simulink library "FIN_MDL"  (R2015a)
settings: Solver=ode45  StartTime=0.0  StopTime=10.0  RelTol=1e-3
undefined symbols (not defined in the file or in its folder): FIN, VAF
libraries: simulink x4
settings Model: Creator=Andrew  LastModifiedBy=Andrew

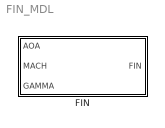
== system FIN_MDL ==
  FIN : Subsystem  mask{FIN=FIN}
      mask prompts: FIN "INPUT  PARAMETERS"

== system FIN_MDL/FIN ==
  AOA : Inport
  MACH : Inport  Port=2
  GAMMA : Inport  Port=3
  Bus Creator : BusCreator  Inputs=5
  FIN_SET_MDL : Subsystem
  FIN : Outport
  wires:
  AOA/1 -> FIN_SET_MDL/1(AOA)
  MACH/1 -> FIN_SET_MDL/2(MACH)
  GAMMA/1 -> FIN_SET_MDL/3(GAMMA)
  FIN_SET_MDL/2(FIN_CN_ALPHA) -> Bus Creator/2  "CN_ALPHA"
  FIN_SET_MDL/1(FIN_CP) -> Bus Creator/1  "CP"
  Bus Creator/1 -> FIN/1
  FIN_SET_MDL/5(FIN_REF_AREA) -> Bus Creator/5  "REF_AREA"
  FIN_SET_MDL/4(FIN_CD) -> Bus Creator/4  "CD"
  FIN_SET_MDL/3(FIN_CN_ALPHA_1) -> Bus Creator/3  "CN_ALPHA_1"

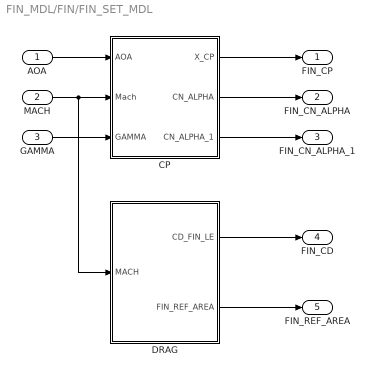
== system FIN_MDL/FIN/FIN_SET_MDL ==
  AOA : Inport
  MACH : Inport  Port=2
  GAMMA : Inport  Port=3
  CP : Subsystem
  DRAG : Subsystem
  FIN_CP : Outport
  FIN_CN_ALPHA : Outport  Port=2
  FIN_CN_ALPHA_1 : Outport  Port=3
  FIN_CD : Outport  Port=4
  FIN_REF_AREA : Outport  Port=5
  wires:
  CP/1(X_CP) -> FIN_CP/1
  CP/2(CN_ALPHA) -> FIN_CN_ALPHA/1
  DRAG/1(CD_FIN_LE) -> FIN_CD/1
  DRAG/2(FIN_REF_AREA) -> FIN_REF_AREA/1
  AOA/1 -> CP/1(AOA)
  GAMMA/1 -> CP/3(GAMMA)
  MACH/1 -> DRAG/1(MACH), CP/2(Mach)
  CP/3(CN_ALPHA_1) -> FIN_CN_ALPHA_1/1

== system FIN_MDL/FIN/FIN_SET_MDL/CP ==
  AOA : Inport
  Mach : Inport  Port=2
  GAMMA : Inport  Port=3
  FIN CP : Subsystem
  SINGLE FIN CN_ALPHA : Subsystem
  TOTAL FIN CN_ALPHA : Subsystem
  X_CP : Outport
  CN_ALPHA : Outport  Port=2
  CN_ALPHA_1 : Outport  Port=3
  wires:
  Mach/1 -> SINGLE FIN CN_ALPHA/1(MACH), FIN CP/1(MACH)
  FIN CP/1(X_CP) -> X_CP/1
  AOA/1 -> SINGLE FIN CN_ALPHA/2(AOA)
  GAMMA/1 -> SINGLE FIN CN_ALPHA/3(GAMMA)
  SINGLE FIN CN_ALPHA/1(CN_ALPHA) -> CN_ALPHA_1/1, TOTAL FIN CN_ALPHA/1(CN_ALPHA_1)
  TOTAL FIN CN_ALPHA/1(CN_ALPHA_FINAL) -> CN_ALPHA/1

== system FIN_MDL/FIN/FIN_SET_MDL/DRAG ==
  MACH : Inport
  Add : Sum
  Constant : Constant  Value=FIN.AREA_REF_DRAG
  Leading Edge : Subsystem
  Trailing Edge : Subsystem
  CD_FIN_LE : Outport
  FIN_REF_AREA : Outport  Port=2
  wires:
  Constant/1 -> FIN_REF_AREA/1
  Add/1 -> CD_FIN_LE/1
  Leading Edge/1(CD_FIN_LE) -> Add/1
  Trailing Edge/1(CD_FIN_TE) -> Add/2
  MACH/1 -> Trailing Edge/1(MACH), Leading Edge/1(MACH)

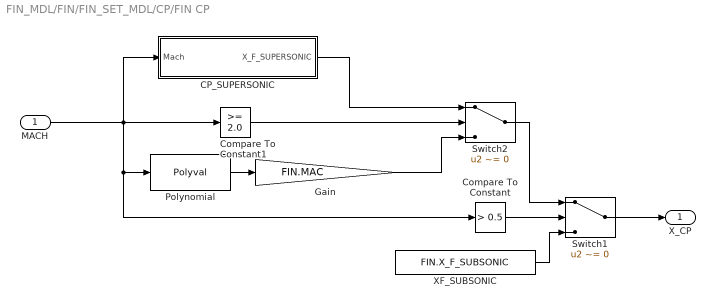
== system FIN_MDL/FIN/FIN_SET_MDL/CP/FIN CP ==
  MACH : Inport
  CP_SUPERSONIC : Subsystem
  Compare To Constant : simulink/Logic and Bit Operations/Compare To Constant  relop=>  const=0.5  OutDataTypeStr=boolean
  Compare To Constant1 : simulink/Logic and Bit Operations/Compare To Constant  relop=>=  const=2.0  OutDataTypeStr=boolean
  Gain : Gain  Gain=FIN.MAC
  Polynomial : Polyval  Coefs=VAF.FIN.MACH_CP_COEFFS
  Switch1 : Switch  Criteria=u2 ~= 0
  Switch2 : Switch  Criteria=u2 ~= 0
  XF_SUBSONIC : FromWorkspace  VariableName=FIN.X_F_SUBSONIC
  X_CP : Outport
  wires:
  Switch1/1 -> X_CP/1
  MACH/1 -> Polynomial/1, Compare To Constant/1, CP_SUPERSONIC/1(Mach), Compare To Constant1/1
  CP_SUPERSONIC/1(X_F_SUPERSONIC) -> Switch2/1
  Switch2/1 -> Switch1/1
  Compare To Constant/1 -> Switch1/2
  Compare To Constant1/1 -> Switch2/2
  XF_SUBSONIC/1 -> Switch1/3
  Polynomial/1 -> Gain/1
  Gain/1 -> Switch2/3

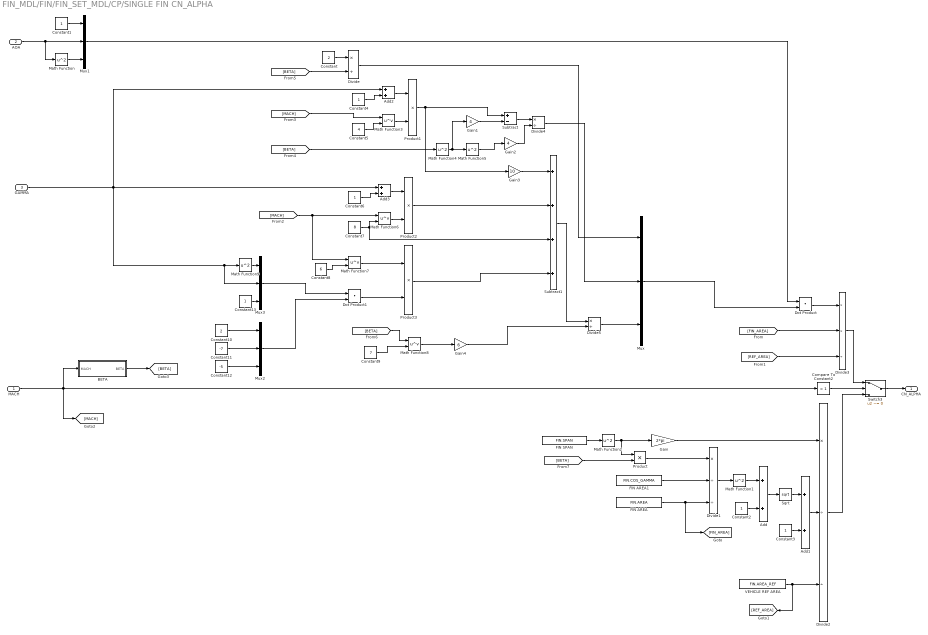
== system FIN_MDL/FIN/FIN_SET_MDL/CP/SINGLE FIN CN_ALPHA ==
  MACH : Inport
  AOA : Inport  Port=2
  GAMMA : Inport  Port=3
  Add{,1..3} (4 alike) : Sum
  BETA : Subsystem
  Compare To Constant2 : simulink/Logic and Bit Operations/Compare To Constant  relop=>  const=1  OutDataTypeStr=boolean
  Constant : Constant  Value=2
  Constant{1..4,6,13} (6 alike) : Constant
  Constant10 : Constant  Value=2
  Constant11 : Constant  Value=-7
  Constant12 : Constant  Value=-5
  Constant5 : Constant  Value=4
  Constant7 : Constant  Value=8
  Constant8 : Constant  Value=6
  Constant9 : Constant  Value=7
  Divide : Product  Inputs=*/
  Divide1 : Product  Inputs=*//
  Divide2 : Product  Inputs=*//
  Divide3 : Product  Inputs=**/
  Divide4 : Product  Inputs=*/
  Divide5 : Product  Inputs=*/
  Dot Product : DotProduct  InputSameDT=on  OutDataTypeStr=Inherit: Inherit via internal rule
  Dot Product1 : DotProduct  InputSameDT=on  OutDataTypeStr=Inherit: Inherit via internal rule
  FIN AREA : FromWorkspace  VariableName=FIN.AREA  SampleTime=0
  FIN AREA1 : FromWorkspace  VariableName=FIN.COS_GAMMA  SampleTime=0
  FIN SPAN : FromWorkspace  VariableName=FIN.SPAN  SampleTime=0
  Gain : Gain  Gain=2*pi
  Gain1 : Gain  Gain=4
  Gain2 : Gain  Gain=4
  Gain3 : Gain  Gain=10
  Gain4 : Gain  Gain=6
  Math Function{,1..2,4..5,9} (6 alike) : Math  Operator=square  SaturateOnIntegerOverflow=on
  Math Function{3,6..8} (4 alike) : Math  Operator=pow  SaturateOnIntegerOverflow=on
  Mux{,1..3} (4 alike) : Mux  Inputs=3
  Product{,1..3} (4 alike) : Product
  Sqrt : Sqrt  SaturateOnIntegerOverflow=on
  Subtract : Sum  Inputs=+-
  Subtract1 : Sum  Inputs=++++
  Switch3 : Switch  Criteria=u2 ~= 0
  VEHICLE REF AREA : FromWorkspace  VariableName=FIN.AREA_REF  SampleTime=0
  CN_ALPHA : Outport
  wires:
  Mux1/1 -> Dot Product/1
  Mux/1 -> Dot Product/2
  Mux2/1 -> Dot Product1/2
  Divide/1 -> Mux/1
  FIN AREA/1 -> [FIN_AREA], Divide1/3
  Product/1 -> Divide1/1
  FIN AREA1/1 -> Divide1/2
  Math Function1/1 -> Add/1
  Divide1/1 -> Math Function1/1
  Constant/1 -> Divide/1
  Math Function2/1 -> Gain/1, Product/1
  FIN SPAN/1 -> Math Function2/1
  Gain3/1 -> Subtract1/1
  Math Function5/1 -> Gain2/1
  Gain/1 -> Divide2/1
  AOA/1 -> Math Function/1, Mux1/2
  Add/1 -> Sqrt/1
  Constant10/1 -> Mux2/1
  Mux3/1 -> Dot Product1/1
  Constant13/1 -> Mux3/3
  Switch3/1 -> CN_ALPHA/1
  Compare To Constant2/1 -> Switch3/2
  Gain2/1 -> Divide4/2
  Math Function4/1 -> Gain1/1, Math Function5/1
  Divide5/1 -> Mux/3
  Constant1/1 -> Mux1/1
  Constant12/1 -> Mux2/3
  Constant9/1 -> Math Function8/2
  Constant4/1 -> Add2/2
  GAMMA/1 -> Mux3/2, Math Function9/1, Add2/1, Add3/1
  VEHICLE REF AREA/1 -> [REF_AREA], Divide2/3
  Add2/1 -> Product1/1
  Math Function3/1 -> Product1/2
  Math Function6/1 -> Product2/2
  Product2/1 -> Subtract1/2
  Constant7/1 -> Subtract1/3, Math Function6/2
  Add3/1 -> Product2/1
  Constant6/1 -> Add3/2
  Dot Product/1 -> Divide3/1
  [FIN_AREA] -> Divide3/2
  [REF_AREA] -> Divide3/3
  Divide3/1 -> Switch3/1
  Math Function9/1 -> Mux3/1
  Add1/1 -> Divide2/2
  Sqrt/1 -> Add1/1
  Constant3/1 -> Add1/2
  Divide2/1 -> Switch3/3
  Gain4/1 -> Divide5/2
  Math Function/1 -> Mux1/3
  Constant2/1 -> Add/2
  Product3/1 -> Subtract1/4
  Math Function7/1 -> Product3/1
  Constant8/1 -> Math Function7/2
  Subtract1/1 -> Divide5/1
  Dot Product1/1 -> Product3/2
  Constant11/1 -> Mux2/2
  Constant5/1 -> Math Function3/2
  Gain1/1 -> Subtract/2
  Product1/1 -> Gain3/1, Subtract/1
  Subtract/1 -> Divide4/1
  Divide4/1 -> Mux/2
  Math Function8/1 -> Gain4/1
  BETA/1(BETA) -> [BETA]
  MACH/1 -> BETA/1(MACH), Compare To Constant2/1, [MACH]
  [MACH] -> Math Function7/1, Math Function6/1
  [MACH] -> Math Function3/1
  [BETA] -> Math Function4/1
  [BETA] -> Divide/2
  [BETA] -> Math Function8/1
  [BETA] -> Product/2

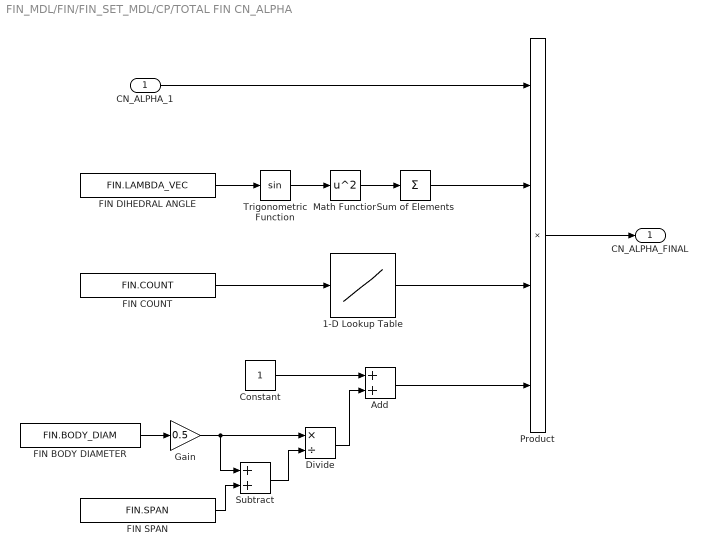
== system FIN_MDL/FIN/FIN_SET_MDL/CP/TOTAL FIN CN_ALPHA ==
  CN_ALPHA_1 : Inport
  1-D Lookup Table : Lookup_n-D  NumberOfTableDimensions=1  BreakpointsForDimension1=FIN.INTERFERE_CORR(:,1)'  Table=FIN.INTERFERE_CORR(:,2)'  InternalRulePriority=Speed  RndMeth=Simplest  InputSameDT=on
  Add : Sum
  Constant : Constant
  Divide : Product  Inputs=*/
  FIN BODY DIAMETER : FromWorkspace  VariableName=FIN.BODY_DIAM  SampleTime=0
  FIN COUNT : FromWorkspace  VariableName=FIN.COUNT  SampleTime=0
  FIN DIHEDRAL ANGLE : FromWorkspace  VariableName=FIN.LAMBDA_VEC  SampleTime=0
  FIN SPAN : FromWorkspace  VariableName=FIN.SPAN  SampleTime=0
  Gain : Gain  Gain=0.5
  Math Function : Math  Operator=square  SaturateOnIntegerOverflow=on
  Product : Product  Inputs=4
  Subtract : Sum
  Sum of Elements : Sum  Inputs=+
  Trigonometric Function : Trigonometry
  CN_ALPHA_FINAL : Outport
  wires:
  FIN DIHEDRAL ANGLE/1 -> Trigonometric Function/1
  Trigonometric Function/1 -> Math Function/1
  Math Function/1 -> Sum of Elements/1
  CN_ALPHA_1/1 -> Product/1
  Sum of Elements/1 -> Product/2
  Product/1 -> CN_ALPHA_FINAL/1
  FIN COUNT/1 -> 1-D Lookup Table/1
  1-D Lookup Table/1 -> Product/3
  Add/1 -> Product/4
  Constant/1 -> Add/1
  FIN BODY DIAMETER/1 -> Gain/1
  Divide/1 -> Add/2
  FIN SPAN/1 -> Subtract/2
  Subtract/1 -> Divide/2
  Gain/1 -> Subtract/1, Divide/1

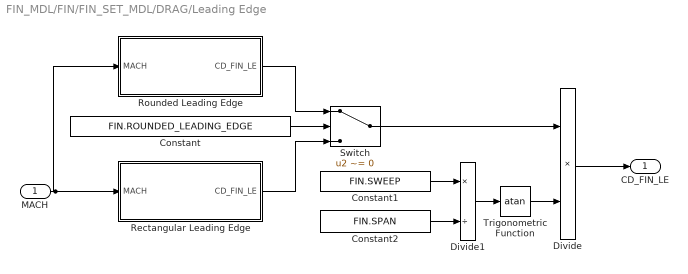
== system FIN_MDL/FIN/FIN_SET_MDL/DRAG/Leading Edge ==
  MACH : Inport
  Constant : Constant  Value=FIN.ROUNDED_LEADING_EDGE
  Constant1 : Constant  Value=FIN.SWEEP
  Constant2 : Constant  Value=FIN.SPAN
  Divide : Product  Inputs=**
  Divide1 : Product  Inputs=*/
  Rectangular Leading Edge : Subsystem
  Rounded Leading Edge : Subsystem
  Switch : Switch  Criteria=u2 ~= 0
  Trigonometric Function : Trigonometry  Operator=atan
  CD_FIN_LE : Outport
  wires:
  Rounded Leading Edge/1(CD_FIN_LE) -> Switch/1
  Rectangular Leading Edge/1(CD_FIN_LE) -> Switch/3
  Constant/1 -> Switch/2
  Constant2/1 -> Divide1/2
  Constant1/1 -> Divide1/1
  Switch/1 -> Divide/1
  Trigonometric Function/1 -> Divide/2
  Divide1/1 -> Trigonometric Function/1
  MACH/1 -> Rounded Leading Edge/1(MACH), Rectangular Leading Edge/1(MACH)
  Divide/1 -> CD_FIN_LE/1

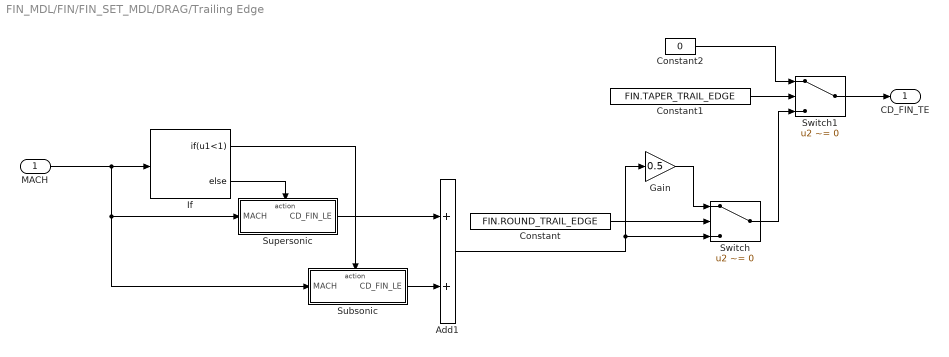
== system FIN_MDL/FIN/FIN_SET_MDL/DRAG/Trailing Edge ==
  MACH : Inport
  Add1 : Sum
  Constant : Constant  Value=FIN.ROUND_TRAIL_EDGE
  Constant1 : Constant  Value=FIN.TAPER_TRAIL_EDGE
  Constant2 : Constant  Value=0
  Gain : Gain  Gain=0.5
  If : If  IfExpression=u1<1
  Subsonic : Subsystem  TreatAsAtomicUnit=on
  Supersonic : Subsystem  TreatAsAtomicUnit=on
  Switch : Switch  Criteria=u2 ~= 0
  Switch1 : Switch  Criteria=u2 ~= 0
  CD_FIN_TE : Outport
  wires:
  If/2 -> Supersonic/Action
  If/1 -> Subsonic/Action
  Subsonic/1(CD_FIN_LE) -> Add1/2
  Supersonic/1(CD_FIN_LE) -> Add1/1
  MACH/1 -> Supersonic/1(MACH), Subsonic/1(MACH), If/1
  Add1/1 -> Gain/1, Switch/3
  Constant/1 -> Switch/2
  Gain/1 -> Switch/1
  Switch/1 -> Switch1/3
  Switch1/1 -> CD_FIN_TE/1
  Constant1/1 -> Switch1/2
  Constant2/1 -> Switch1/1

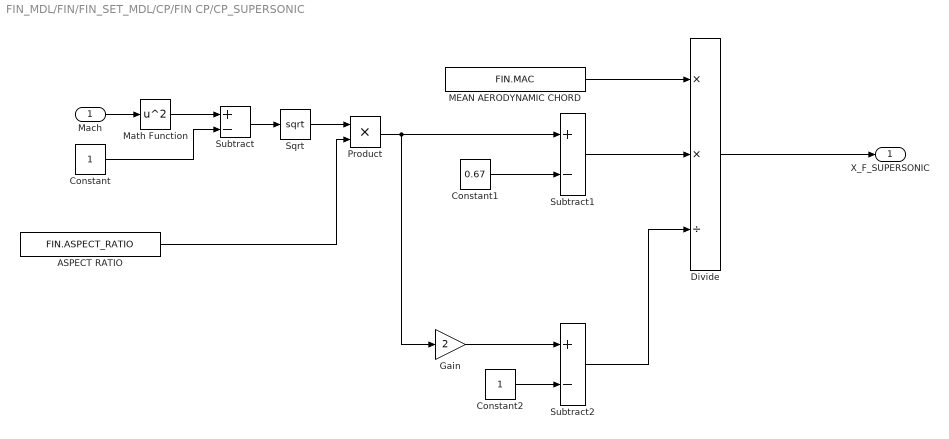
== system FIN_MDL/FIN/FIN_SET_MDL/CP/FIN CP/CP_SUPERSONIC ==
  Mach : Inport
  ASPECT RATIO : FromWorkspace  VariableName=FIN.ASPECT_RATIO
  Constant : Constant
  Constant1 : Constant  Value=0.67
  Constant2 : Constant
  Divide : Product  Inputs=**/
  Gain : Gain  Gain=2
  MEAN AERODYNAMIC CHORD : FromWorkspace  VariableName=FIN.MAC
  Math Function : Math  Operator=square  SaturateOnIntegerOverflow=on
  Product : Product
  Sqrt : Sqrt  SaturateOnIntegerOverflow=on
  Subtract : Sum  Inputs=+-
  Subtract1 : Sum  Inputs=+-
  Subtract2 : Sum  Inputs=+-
  X_F_SUPERSONIC : Outport
  wires:
  Mach/1 -> Math Function/1
  Constant/1 -> Subtract/2
  Math Function/1 -> Subtract/1
  Subtract/1 -> Sqrt/1
  Sqrt/1 -> Product/1
  ASPECT RATIO/1 -> Product/2
  Product/1 -> Gain/1, Subtract1/1
  Constant1/1 -> Subtract1/2
  Constant2/1 -> Subtract2/2
  Subtract1/1 -> Divide/2
  Subtract2/1 -> Divide/3
  Divide/1 -> X_F_SUPERSONIC/1
  Gain/1 -> Subtract2/1
  MEAN AERODYNAMIC CHORD/1 -> Divide/1

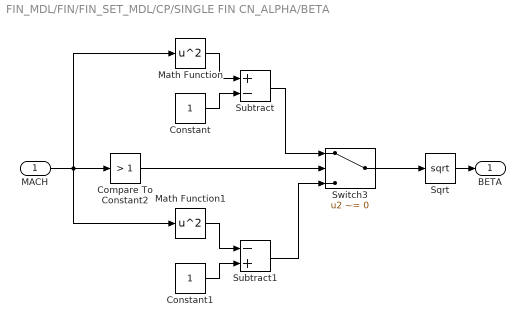
== system FIN_MDL/FIN/FIN_SET_MDL/CP/SINGLE FIN CN_ALPHA/BETA ==
  MACH : Inport
  Compare To Constant2 : simulink/Logic and Bit Operations/Compare To Constant  relop=>  const=1  OutDataTypeStr=boolean
  Constant : Constant
  Constant1 : Constant
  Math Function : Math  Operator=square  SaturateOnIntegerOverflow=on
  Math Function1 : Math  Operator=square  SaturateOnIntegerOverflow=on
  Sqrt : Sqrt  SaturateOnIntegerOverflow=on
  Subtract : Sum  Inputs=+-
  Subtract1 : Sum  Inputs=-+
  Switch3 : Switch  Criteria=u2 ~= 0
  BETA : Outport
  wires:
  Switch3/1 -> Sqrt/1
  Subtract1/1 -> Switch3/3
  Constant1/1 -> Subtract1/2
  Math Function1/1 -> Subtract1/1
  Constant/1 -> Subtract/2
  Subtract/1 -> Switch3/1
  Math Function/1 -> Subtract/1
  MACH/1 -> Math Function/1, Math Function1/1, Compare To Constant2/1
  Sqrt/1 -> BETA/1
  Compare To Constant2/1 -> Switch3/2

== system FIN_MDL/FIN/FIN_SET_MDL/DRAG/Leading Edge/Rectangular Leading Edge ==
  MACH : Inport
  Add1 : Sum
  If : If  IfExpression=u1<1
  Subsonic : Subsystem  TreatAsAtomicUnit=on
  Supersonic : Subsystem  TreatAsAtomicUnit=on
  CD_FIN_LE : Outport
  wires:
  MACH/1 -> If/1, Subsonic/1(MACH), Supersonic/1(MACH)
  Supersonic/1(CD_FIN_LE) -> Add1/1
  Subsonic/1(CD_FIN_LE) -> Add1/2
  If/1 -> Subsonic/Action
  If/2 -> Supersonic/Action
  Add1/1 -> CD_FIN_LE/1

== system FIN_MDL/FIN/FIN_SET_MDL/DRAG/Leading Edge/Rounded Leading Edge ==
  MACH : Inport
  Add1 : Sum  Inputs=+++
  If : If  IfExpression=u1<0.9  ElseIfExpressions=u1>1
  Subsonic : Subsystem  TreatAsAtomicUnit=on
  Supersonic : Subsystem  TreatAsAtomicUnit=on
  Transonic : Subsystem  TreatAsAtomicUnit=on
  CD_FIN_LE : Outport
  wires:
  Add1/1 -> CD_FIN_LE/1
  If/3 -> Transonic/Action
  If/1 -> Subsonic/Action
  If/2 -> Supersonic/Action
  Subsonic/1(CD_FIN_LE) -> Add1/3
  Transonic/1(CD_FIN_LE) -> Add1/1
  Supersonic/1(CD_FIN_LE) -> Add1/2
  MACH/1 -> Transonic/1(MACH), Supersonic/1(MACH), Subsonic/1(MACH), If/1

== system FIN_MDL/FIN/FIN_SET_MDL/DRAG/Trailing Edge/Subsonic ==
  note: CD_LE = 1 + M^2/4 + M^4 / 40
  MACH : Inport
  Action Port : ActionPort
  Constant : Constant  Value=0.12
  Gain : Gain  Gain=0.13
  Math Function : Math  Operator=square  SaturateOnIntegerOverflow=on
  Subtract : Sum
  CD_FIN_LE : Outport
  wires:
  Gain/1 -> Subtract/1
  Subtract/1 -> CD_FIN_LE/1
  MACH/1 -> Math Function/1
  Math Function/1 -> Gain/1
  Constant/1 -> Subtract/2

== system FIN_MDL/FIN/FIN_SET_MDL/DRAG/Trailing Edge/Supersonic ==
  MACH : Inport
  Action Port : ActionPort
  Gain : Gain  Gain=0.25
  Math Function : Math  Operator=reciprocal  SaturateOnIntegerOverflow=on
  CD_FIN_LE : Outport
  wires:
  Math Function/1 -> Gain/1
  MACH/1 -> Math Function/1
  Gain/1 -> CD_FIN_LE/1

== system FIN_MDL/FIN/FIN_SET_MDL/DRAG/Leading Edge/Rectangular Leading Edge/Subsonic ==
  note: CD_LE = 1 + M^2/4 + M^4 / 40
  MACH : Inport
  Action Port : ActionPort
  Constant : Constant
  Gain : Gain  Gain=0.25
  Gain1 : Gain  Gain=1/40
  Math Function : Math  Operator=square  SaturateOnIntegerOverflow=on
  Math Function1 : Math  Operator=square  SaturateOnIntegerOverflow=on
  Subtract : Sum  Inputs=+++
  CD_FIN_LE : Outport
  wires:
  Math Function/1 -> Gain/1, Math Function1/1
  MACH/1 -> Math Function/1
  Subtract/1 -> CD_FIN_LE/1
  Gain/1 -> Subtract/1
  Math Function1/1 -> Gain1/1
  Gain1/1 -> Subtract/2
  Constant/1 -> Subtract/3

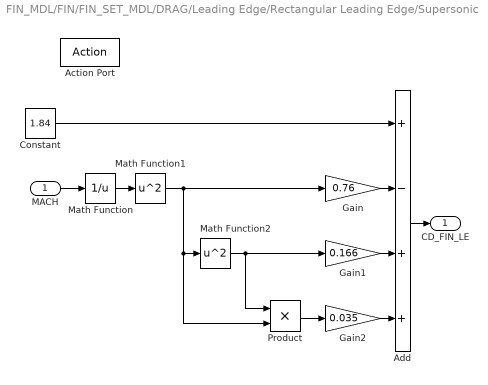
== system FIN_MDL/FIN/FIN_SET_MDL/DRAG/Leading Edge/Rectangular Leading Edge/Supersonic ==
  MACH : Inport
  Action Port : ActionPort
  Add : Sum  Inputs=+-++
  Constant : Constant  Value=1.84
  Gain : Gain  Gain=0.76
  Gain1 : Gain  Gain=0.166
  Gain2 : Gain  Gain=0.035
  Math Function : Math  Operator=reciprocal  SaturateOnIntegerOverflow=on
  Math Function1 : Math  Operator=square  SaturateOnIntegerOverflow=on
  Math Function2 : Math  Operator=square  SaturateOnIntegerOverflow=on
  Product : Product
  CD_FIN_LE : Outport
  wires:
  Gain/1 -> Add/2
  Constant/1 -> Add/1
  Add/1 -> CD_FIN_LE/1
  MACH/1 -> Math Function/1
  Math Function/1 -> Math Function1/1
  Math Function2/1 -> Gain1/1, Product/1
  Math Function1/1 -> Math Function2/1, Product/2, Gain/1
  Product/1 -> Gain2/1
  Gain1/1 -> Add/3
  Gain2/1 -> Add/4

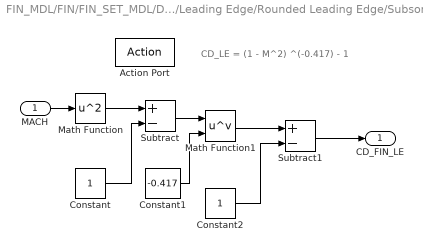
== system FIN_MDL/FIN/FIN_SET_MDL/DRAG/Leading Edge/Rounded Leading Edge/Subsonic ==
  note: CD_LE = (1 - M^2) ^(-0.417) - 1
  MACH : Inport
  Action Port : ActionPort
  Constant : Constant
  Constant1 : Constant  Value=-0.417
  Constant2 : Constant
  Math Function : Math  Operator=square  SaturateOnIntegerOverflow=on
  Math Function1 : Math  Operator=pow  SaturateOnIntegerOverflow=on
  Subtract : Sum  Inputs=+-
  Subtract1 : Sum  Inputs=+-
  CD_FIN_LE : Outport
  wires:
  MACH/1 -> Math Function/1
  Math Function/1 -> Subtract/1
  Constant/1 -> Subtract/2
  Subtract/1 -> Math Function1/1
  Constant1/1 -> Math Function1/2
  Math Function1/1 -> Subtract1/1
  Constant2/1 -> Subtract1/2
  Subtract1/1 -> CD_FIN_LE/1

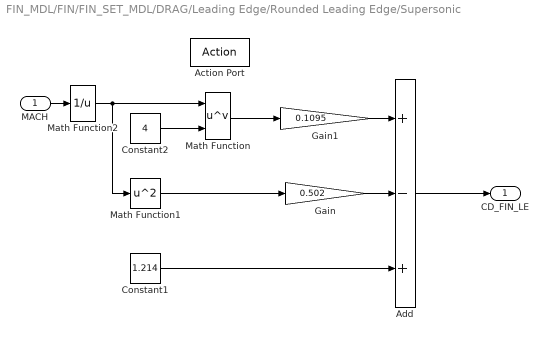
== system FIN_MDL/FIN/FIN_SET_MDL/DRAG/Leading Edge/Rounded Leading Edge/Supersonic ==
  MACH : Inport
  Action Port : ActionPort
  Add : Sum  Inputs=+-+
  Constant1 : Constant  Value=1.214
  Constant2 : Constant  Value=4
  Gain : Gain  Gain=0.502
  Gain1 : Gain  Gain=0.1095
  Math Function : Math  Operator=pow  SaturateOnIntegerOverflow=on
  Math Function1 : Math  Operator=square  SaturateOnIntegerOverflow=on
  Math Function2 : Math  Operator=reciprocal  SaturateOnIntegerOverflow=on
  CD_FIN_LE : Outport
  wires:
  Constant1/1 -> Add/3
  MACH/1 -> Math Function2/1
  Math Function2/1 -> Math Function1/1, Math Function/1
  Math Function1/1 -> Gain/1
  Gain/1 -> Add/2
  Constant2/1 -> Math Function/2
  Add/1 -> CD_FIN_LE/1
  Math Function/1 -> Gain1/1
  Gain1/1 -> Add/1

== system FIN_MDL/FIN/FIN_SET_MDL/DRAG/Leading Edge/Rounded Leading Edge/Transonic ==
  MACH : Inport
  Action Port : ActionPort
  Add : Sum  Inputs=-+
  Add1 : Sum  Inputs=+-
  Constant : Constant
  Constant1 : Constant  Value=0.9
  Gain : Gain  Gain=1.785
  CD_FIN_LE : Outport
  wires:
  Add/1 -> CD_FIN_LE/1
  Constant/1 -> Add/1
  MACH/1 -> Add1/1
  Constant1/1 -> Add1/2
  Add1/1 -> Gain/1
  Gain/1 -> Add/2
